simulink model "Eulers"  (R2024b)
settings: Solver=FixedStepAuto  StartTime=0.0  StopTime=10  FixedStep=1e-3  RelTol=1e-3
libraries: shared6dof x1, simulink x1
settings Model: PacingRate=0.010000  Creator=cpero  LastModifiedBy=cpero

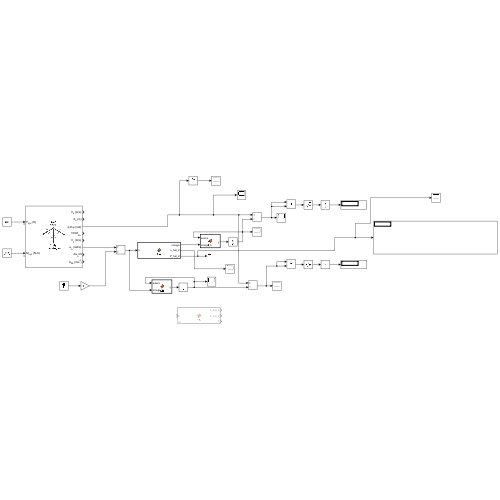
[thumbnail: Simulink's stored preview of the top-level diagram]
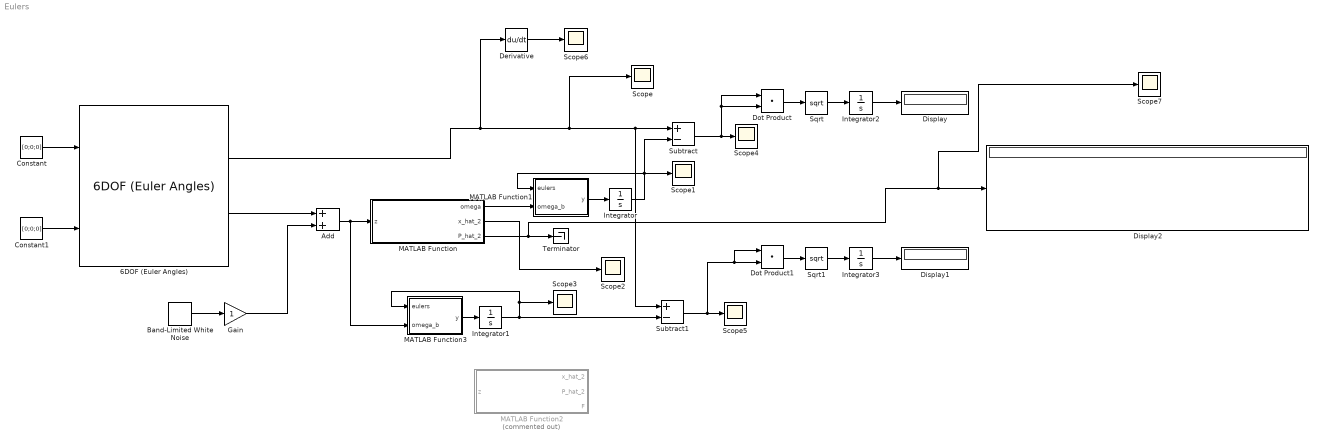
== system Eulers ==
  6DOF (Euler Angles) : shared6dof/6DOF (Euler Angles)  units=Metric (MKS)  mtype=Fixed  rep=Euler Angles  xme_0=[0 0 0]  Vm_0=[0 0 0]  eul_0=[0 0 0]  pm_0=[0.01 0 0]  mass_0=1.0  mass_e=0.5  mass_f=2.0  inertia=eye(3)  inertia_e=eye(3)  inertia_f=2*eye(3)  k_quat=1.0  vre_flag=on  abi_flag=off  aMode=0  xme_statename=''  Vm_statename=''  eul_statename=''  quat_statename=''  pm_statename=''  mass_statename=''
  Add : Sum
  Band-Limited White Noise : simulink/Sources/Band-Limited White Noise  Cov=[1e-6 1e-6 1e-6]  Ts=0.001  seed=[1 2 3]
  Constant : Constant  Value=[0;0;0]
  Constant1 : Constant  Value=[0;0;0]
  Derivative : Derivative
  Display : Display
  Display1 : Display
  Display2 : Display
  Dot Product : DotProduct  OutDataTypeStr=Inherit: Inherit via internal rule
  Dot Product1 : DotProduct  OutDataTypeStr=Inherit: Inherit via internal rule
  Gain : Gain
  Integrator : Integrator  InitialCondition=[0;0;0];
  Integrator1 : Integrator  InitialCondition=[0;0;0];
  Integrator2 : Integrator
  Integrator3 : Integrator
  MATLAB Function : MATLAB Function  TreatAsAtomicUnit=on
  MATLAB Function1 : MATLAB Function  TreatAsAtomicUnit=on
  MATLAB Function2 : MATLAB Function  Commented=on  TreatAsAtomicUnit=on
  MATLAB Function3 : MATLAB Function  TreatAsAtomicUnit=on
  Scope{,1..7} (8 alike) : Scope
  Sqrt : Sqrt
  Sqrt1 : Sqrt
  Subtract : Sum  Inputs=+-
  Subtract1 : Sum  Inputs=+-
  Terminator : Terminator
  wires:
  Band-Limited White Noise/1 -> Gain/1
  Gain/1 -> Add/2
  Constant/1 -> 6DOF (Euler Angles)/1
  Constant1/1 -> 6DOF (Euler Angles)/2
  6DOF (Euler Angles)/6 -> Add/1
  Subtract/1 -> Dot Product/1, Dot Product/2, Scope4/1
  MATLAB Function/2(x_hat_2) -> Scope2/1
  MATLAB Function1/1(y) -> Integrator/1
  Integrator/1 -> Scope1/1, Subtract/2, MATLAB Function1/1(eulers)
  6DOF (Euler Angles)/3 -> Scope/1, Subtract1/1, Subtract/1, Derivative/1
  MATLAB Function/3(P_hat_2) -> Scope7/1, Display2/1, Terminator/1
  MATLAB Function/1(omega) -> MATLAB Function1/2(omega_b)
  Integrator1/1 -> Subtract1/2, Scope3/1, MATLAB Function3/1(eulers)
  MATLAB Function3/1(y) -> Integrator1/1
  Dot Product/1 -> Sqrt/1
  Sqrt/1 -> Integrator2/1
  Dot Product1/1 -> Sqrt1/1
  Subtract1/1 -> Dot Product1/1, Dot Product1/2, Scope5/1
  Sqrt1/1 -> Integrator3/1
  Integrator2/1 -> Display/1
  Integrator3/1 -> Display1/1
  Derivative/1 -> Scope6/1
  Add/1 -> MATLAB Function3/2(omega_b), MATLAB Function/1(z)

== matlab function Eulers/MATLAB Function1 ==
  data: eulers input; y output; omega_b input
function y = fcn(eulers, omega_b)

phi = eulers(1);
theta = eulers(2);
psi = eulers(3);

L = [1 sin(phi)*tan(theta) cos(phi)*tan(theta);
     0 cos(phi) -sin(phi);
     0 sin(phi)*sec(theta) cos(phi)*sec(theta)];

y = L*omega_b;

== matlab function Eulers/MATLAB Function ==
  settings: updateMethod=DISCRETE
  data: omega output; z input; x_hat_2 output; P_hat_2 output
function [omega, x_hat_2, P_hat_2] = fcn(z)

persistent x_hat_2_prior P_hat_2_prior

dt = 1e-3;

if isempty(x_hat_2_prior)
    x_hat_2_prior = [0.01;0;0;0;0;0];
    P_hat_2_prior = kron(diag([1e-3,1e-2]),eye(3));
end

A = [1 dt;
     0 1];
F = kron(A,eye(3));
H = [eye(3) zeros(3)];
Q = zeros(6);
R = 1e2*eye(3);

%Predict
x_hat_1 = F*x_hat_2_prior;
P_hat_1 = F*P_hat_2_prior*F' + Q;

%Update
y = z - H*x_hat_1;
S = H*P_hat_1*H' + R;
K = P_hat_1*H'*inv(S);
x_hat_2 = x_hat_1 + K*y;
P_hat_2 = (eye(6) - K*H)*P_hat_1;

omega = x_hat_2(1:3);
x_hat_2_prior = x_hat_2;
P_hat_2_prior = P_hat_2;

== matlab function Eulers/MATLAB Function2 ==
  settings: updateMethod=DISCRETE
  data: z input; x_hat_2 output; P_hat_2 output; F output
function [x_hat_2, P_hat_2, F] = fcn(z)

persistent x_hat_2_prior P_hat_2_prior

if isempty(x_hat_2_prior)
    x_hat_2_prior = [0;0;0;0.2;0;0];
    P_hat_2_prior = eye(6);
end

dt = 1e-3;

%A = [1 dt;
%     0 1];
%F = kron(A,eye(3));
H = [zeros(3) eye(3)];
Q = zeros(6);
R = eye(3);

phi = x_hat_2_prior(1);
theta = x_hat_2_prior(2);
psi = x_hat_2_prior(3);

p = z(1);
q = z(2);
r = z(3);

f1 = [1 + dt*(q*tan(theta)*cos(phi)-r*tan(theta)*sin(phi)); dt*(q*cos(phi)*sec(theta)^2-r*sin(phi)*sec(theta)^2); 0];
f2 = [dt*(-1*sin(phi)-r*cos(phi)); 1; 0];
f3 = [dt*(q*sec(theta)*cos(phi)-r*sec(theta)*sin(phi)); dt*(q*sin(phi)*tan(theta)*sec(theta)+r*cos(phi)*tan(theta)*sec(theta)); 1];
F = [[f1 f2 f3],zeros(3);
     zeros(3), eye(3)];

%Predict
x_hat_1 = [x_hat_2_prior(1:3) + dt*z; z];
P_hat_1 = F*P_hat_2_prior*F' + Q;

%Update
y = z - H*x_hat_1;
S = H*P_hat_1*H' + R;
K = P_hat_1*H'*inv(S);
x_hat_2 = x_hat_1 + K*y;
P_hat_2 = (eye(6) - K*H)*P_hat_1;

x_hat_2_prior = x_hat_2;
P_hat_2_prior = P_hat_2;

== matlab function Eulers/MATLAB Function3 ==
  data: eulers input; y output; omega_b input
function y = fcn(eulers, omega_b)

phi = eulers(1);
theta = eulers(2);
psi = eulers(3);

L = [1 sin(phi)*tan(theta) cos(phi)*tan(theta);
     0 cos(phi) -sin(phi);
     0 sin(phi)*sec(theta) cos(phi)*sec(theta)];

y = L*omega_b;
